simulink model "pulsar_channeliser"  (R2012b)
settings: Solver=ode45  StartTime=0.0  StopTime=450e6  RelTol=1e-3
undefined symbols (not defined in the file): pfb_coeff_gen_calc, sigbuilder_block
libraries: xbsIndex_r4 x10677, casper_library_delays x128, casper_library_misc x45, simulink x17, dspsigops x12, xps_library x9, casper_library_flow_control x4, casper_library_pfbs x2
(part 5 of 105)

== system pulsar_channeliser/frame_counter ==
  note: Knowing the band select will tell us how many
      | channels we actually have to put through,
      | and hence how many words need to be read
      | out of the FIFO at once.
      | Explanation:
      | 0 (16 chans) - 512 words, 64 frames
      | 1 (14 chans) - 518 words, 74 frames
      | 2 (12 chans) - 516 words, 86 frames
      | 3 (10 chans) - 515 words, 103 frames
      | 4 (8 chans) - 512 words, 128 frames
      | 5 (6 chans) - 513 words, 171 frames
      | 6 (4 chans) - 512 words, 256 frames
      | 7 (2 chans) - 512 words, 512 frames
  note: 31-bit counter, along with 10-bit number below, would make a 41-bit
      | output but since the number is 10-bit only to accommodate 512, it'll
      | never actually get to 41 bits. Just 40. So I'll chop the top one off.
  reset : Inport
  dv : Inport  Port=2
  band_select : Inport  Port=3
  Constant10 : xbsIndex_r4/Constant  const=86  gui_display_data_type=Fixed-point  arith_type=Unsigned  n_bits=10  bin_pt=0  preci_type=Single  exp_width=8  frac_width=24  explicit_period=on  period=1  equ=P=C  opselect=C  inp2=PCIN>>17  opr=+  inp1=P  carry=CIN  dbl_ovrd=off  block_type=constant
  Constant11 : xbsIndex_r4/Constant  const=103  gui_display_data_type=Fixed-point  arith_type=Unsigned  n_bits=10  bin_pt=0  preci_type=Single  exp_width=8  frac_width=24  explicit_period=on  period=1  equ=P=C  opselect=C  inp2=PCIN>>17  opr=+  inp1=P  carry=CIN  dbl_ovrd=off  block_type=constant
  Constant12 : xbsIndex_r4/Constant  const=171  gui_display_data_type=Fixed-point  arith_type=Unsigned  n_bits=10  bin_pt=0  preci_type=Single  exp_width=8  frac_width=24  explicit_period=on  period=1  equ=P=C  opselect=C  inp2=PCIN>>17  opr=+  inp1=P  carry=CIN  dbl_ovrd=off  block_type=constant
  Constant13 : xbsIndex_r4/Constant  const=128  gui_display_data_type=Fixed-point  arith_type=Unsigned  n_bits=10  bin_pt=0  preci_type=Single  exp_width=8  frac_width=24  explicit_period=on  period=1  equ=P=C  opselect=C  inp2=PCIN>>17  opr=+  inp1=P  carry=CIN  dbl_ovrd=off  block_type=constant
  Constant14 : xbsIndex_r4/Constant  const=256  gui_display_data_type=Fixed-point  arith_type=Unsigned  n_bits=10  bin_pt=0  preci_type=Single  exp_width=8  frac_width=24  explicit_period=on  period=1  equ=P=C  opselect=C  inp2=PCIN>>17  opr=+  inp1=P  carry=CIN  dbl_ovrd=off  block_type=constant
  Constant15 : xbsIndex_r4/Constant  const=512  gui_display_data_type=Fixed-point  arith_type=Unsigned  n_bits=10  bin_pt=0  preci_type=Single  exp_width=8  frac_width=24  explicit_period=on  period=1  equ=P=C  opselect=C  inp2=PCIN>>17  opr=+  inp1=P  carry=CIN  dbl_ovrd=off  block_type=constant
  Constant7 : xbsIndex_r4/Constant  const=64  gui_display_data_type=Fixed-point  arith_type=Unsigned  n_bits=10  bin_pt=0  preci_type=Single  exp_width=8  frac_width=24  explicit_period=on  period=1  equ=P=C  opselect=C  inp2=PCIN>>17  opr=+  inp1=P  carry=CIN  dbl_ovrd=off  block_type=constant
  Constant9 : xbsIndex_r4/Constant  const=74  gui_display_data_type=Fixed-point  arith_type=Unsigned  n_bits=10  bin_pt=0  preci_type=Single  exp_width=8  frac_width=24  explicit_period=on  period=1  equ=P=C  opselect=C  inp2=PCIN>>17  opr=+  inp1=P  carry=CIN  dbl_ovrd=off  block_type=constant
  Counter : xbsIndex_r4/Counter  cnt_type=Free Running  cnt_to=Inf  operation=Up  start_count=0  cnt_by_val=1  arith_type=Unsigned  n_bits=31  bin_pt=0  load_pin=off  rst=on  en=on  explicit_period=on  period=1  dbl_ovrd=off  use_behavioral_HDL=off  implementation=Fabric  block_type=counter
  Mult : xbsIndex_r4/Mult  precision=Full  arith_type="Signed  (2's comp)"  n_bits=16  bin_pt=14  quantization=Truncate  overflow=Wrap  en=off  latency=3  dbl_ovrd=off  use_behavioral_HDL=off  opt=Speed  use_embedded=on  optimum_pipeline=off  pipeline=on  use_rpm=on  placement_style=Triangular  block_type=mult
  Mux1 : xbsIndex_r4/Mux  inputs=8  en=off  latency=0  precision=Full  arith_type=Unsigned  n_bits=16  bin_pt=14  quantization=Truncate  overflow=Wrap  dbl_ovrd=off  block_type=mux
  Slice : xbsIndex_r4/Slice  nbits=40  boolean_output=off  mode=Lower Bit Location + Width  bit1=0  base1=MSB of Input  bit0=0  base0=LSB of Input  dbl_ovrd=off  block_type=slice
  Slice1 : xbsIndex_r4/Slice  nbits=3  boolean_output=off  mode=Upper Bit Location + Width  bit1=0  base1=MSB of Input  bit0=1  base0=LSB of Input  dbl_ovrd=off  block_type=slice
  edge_detect1 : casper_library_misc/edge_detect  edge=Rising  polarity=Active High  x_in=[0 0.08 0.08 0.16 0.16 0.24 0.24 0.32 0.32 0.4]  y_in="[-1 -1  1  1  1  1  1  1  1  1]"  x_out=[0.6 0.68 0.68 0.76 0.76 0.84 0.84 0.92 0.92 1]  y_out="[-1 -1  1  1 -1 -1 -1 -1 -1 -1]"
  frame_count : Outport
  wires:
  dv/1 -> edge_detect1/1
  reset/1 -> Counter/1
  edge_detect1/1 -> Counter/2
  Slice1/1 -> Mux1/1
  Constant7/1 -> Mux1/2
  Constant9/1 -> Mux1/3
  Constant10/1 -> Mux1/4
  Constant11/1 -> Mux1/5
  Constant12/1 -> Mux1/7
  band_select/1 -> Slice1/1
  Constant13/1 -> Mux1/6
  Constant14/1 -> Mux1/8
  Constant15/1 -> Mux1/9
  Mux1/1 -> Mult/2
  Counter/1 -> Mult/1
  Mult/1 -> Slice/1
  Slice/1 -> frame_count/1

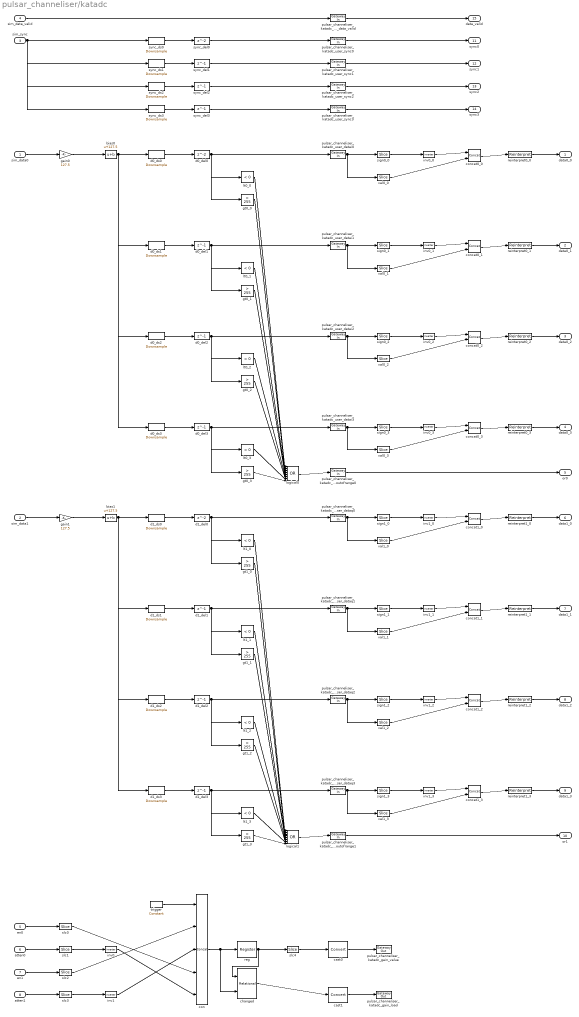
== system pulsar_channeliser/katadc ==
  sim_data0 : Inport
  sim_data1 : Inport  Port=2
  sim_sync : Inport  Port=3
  sim_data_valid : Inport  Port=4
  en0 : Inport  Port=5
  atten0 : Inport  Port=6
  en1 : Inport  Port=7
  atten1 : Inport  Port=8
  bias0 : Bias  Bias=127.5  SaturateOnIntegerOverflow=on
  bias1 : Bias  Bias=127.5  SaturateOnIntegerOverflow=on
  cast0 : xbsIndex_r4/Convert  gui_display_data_type=Fixed-point  arith_type=Unsigned  n_bits=14  bin_pt=0  float_type=Single  exp_bits=8  fraction_bits=24  quantization=Truncate  overflow=Wrap  en=off  latency=0  dbl_ovrd=off  pipeline=off  block_type=convert
      settings: block_version=11.4
  cast1 : xbsIndex_r4/Convert  gui_display_data_type=Fixed-point  arith_type=Boolean  n_bits=16  bin_pt=14  float_type=Single  exp_bits=8  fraction_bits=24  quantization=Truncate  overflow=Wrap  en=off  latency=0  dbl_ovrd=off  pipeline=off  block_type=convert
      settings: block_version=11.4
  changed : xbsIndex_r4/Relational  mode=a!=b  en=off  latency=1  dbl_ovrd=off  block_type=relational
  con : xbsIndex_r4/Concat  num_inputs=5  dbl_ovrd=off  block_type=concat
  concat0_{0..3} (4 alike) : xbsIndex_r4/Concat  num_inputs=2  dbl_ovrd=off  block_type=concat
  concat1_{0..3} (4 alike) : xbsIndex_r4/Concat  num_inputs=2  dbl_ovrd=off  block_type=concat
  d0_del0 : Delay  InputProcessing=Inherited
  d0_del1 : Delay  DelayLength=1  InputProcessing=Inherited
  d0_del2 : Delay  DelayLength=1  InputProcessing=Inherited
  d0_del3 : Delay  DelayLength=1  InputProcessing=Inherited
  d0_ds0 : dspsigops/Downsample  N=4  phase=0  RateOptions=Allow multirate processing  smode=Allow multirate  fmode=Maintain input frame size  ic=0
  d0_ds1 : dspsigops/Downsample  N=4  phase=1  RateOptions=Allow multirate processing  smode=Allow multirate  fmode=Maintain input frame size  ic=0
  d0_ds2 : dspsigops/Downsample  N=4  phase=2  RateOptions=Allow multirate processing  smode=Allow multirate  fmode=Maintain input frame size  ic=0
  d0_ds3 : dspsigops/Downsample  N=4  phase=3  RateOptions=Allow multirate processing  smode=Allow multirate  fmode=Maintain input frame size  ic=0
  d1_del0 : Delay  InputProcessing=Inherited
  d1_del1 : Delay  DelayLength=1  InputProcessing=Inherited
  d1_del2 : Delay  DelayLength=1  InputProcessing=Inherited
  d1_del3 : Delay  DelayLength=1  InputProcessing=Inherited
  d1_ds0 : dspsigops/Downsample  N=4  phase=0  RateOptions=Allow multirate processing  smode=Allow multirate  fmode=Maintain input frame size  ic=0
  d1_ds1 : dspsigops/Downsample  N=4  phase=1  RateOptions=Allow multirate processing  smode=Allow multirate  fmode=Maintain input frame size  ic=0
  d1_ds2 : dspsigops/Downsample  N=4  phase=2  RateOptions=Allow multirate processing  smode=Allow multirate  fmode=Maintain input frame size  ic=0
  d1_ds3 : dspsigops/Downsample  N=4  phase=3  RateOptions=Allow multirate processing  smode=Allow multirate  fmode=Maintain input frame size  ic=0
  gain0 : Gain  Gain=127.5  SaturateOnIntegerOverflow=on  OutDataTypeStr=Inherit: Same as input  ParamDataTypeStr=Inherit: Same as input
  gain1 : Gain  Gain=127.5  SaturateOnIntegerOverflow=on  OutDataTypeStr=Inherit: Same as input  ParamDataTypeStr=Inherit: Same as input
  gt0_{0..3} (4 alike) : simulink/Logic and Bit Operations/Compare To Constant  relop=>  const=255  OutDataTypeStr=boolean  ZeroCross=off
  gt1_{0..3} (4 alike) : simulink/Logic and Bit Operations/Compare To Constant  relop=>  const=255  OutDataTypeStr=boolean  ZeroCross=off
  inv0 : xbsIndex_r4/Inverter  en=off  latency=0  dbl_ovrd=off  block_type=inv
      settings: block_version=11.4
  inv0_{0..3} (4 alike) : xbsIndex_r4/Inverter  en=off  latency=0  dbl_ovrd=off  block_type=inv
      settings: block_version=11.4
  inv1 : xbsIndex_r4/Inverter  en=off  latency=0  dbl_ovrd=off  block_type=inv
      settings: block_version=11.4
  inv1_{0..3} (4 alike) : xbsIndex_r4/Inverter  en=off  latency=0  dbl_ovrd=off  block_type=inv
      settings: block_version=11.4
  logical0 : Logic  Operator=OR  Inputs=8
  logical1 : Logic  Operator=OR  Inputs=8
  lt0_{0..3} (4 alike) : simulink/Logic and Bit Operations/Compare To Constant  relop=<  const=0  OutDataTypeStr=boolean  ZeroCross=off
  lt1_{0..3} (4 alike) : simulink/Logic and Bit Operations/Compare To Constant  relop=<  const=0  OutDataTypeStr=boolean  ZeroCross=off
  pulsar_channeliser_katadc_gain_load : xbsIndex_r4/Gateway Out  inherit_from_input=off  hdl_port=on  timing_constraint=None  locs_specified=off  LOCs={}  UseAsDAC=off  DACChannel='1'  block_type=gatewayout
  pulsar_channeliser_katadc_gain_value : xbsIndex_r4/Gateway Out  inherit_from_input=off  hdl_port=on  timing_constraint=None  locs_specified=off  LOCs={}  UseAsDAC=off  DACChannel='1'  block_type=gatewayout
  pulsar_channeliser_katadc_user_data_valid : xbsIndex_r4/Gateway In  gui_display_data_type=Fixed-point  arith_type=Boolean  n_bits=16  bin_pt=14  preci_type=Single  exp_width=8  frac_width=24  quantization="Round  (unbiased: +/- Inf)"  overflow=Saturate  period=1  dbl_ovrd=off  timing_constraint=None  locs_specified=off  LOCs={}  UseAsADC=off  ADCChannel='1'  inherit_from_input=off  hdl_port=on  block_type=gatewayin
  pulsar_channeliser_katadc_user_datai{0..3} (4 alike) : xbsIndex_r4/Gateway In  gui_display_data_type=Fixed-point  arith_type=Unsigned  n_bits=8  bin_pt=0  preci_type=Single  exp_width=8  frac_width=24  quantization="Round  (unbiased: +/- Inf)"  overflow=Saturate  period=1  dbl_ovrd=off  timing_constraint=None  locs_specified=off  LOCs={}  UseAsADC=off  ADCChannel='1'  inherit_from_input=off  hdl_port=on  block_type=gatewayin
  pulsar_channeliser_katadc_user_dataq{0..3} (4 alike) : xbsIndex_r4/Gateway In  gui_display_data_type=Fixed-point  arith_type=Unsigned  n_bits=8  bin_pt=0  preci_type=Single  exp_width=8  frac_width=24  quantization="Round  (unbiased: +/- Inf)"  overflow=Saturate  period=1  dbl_ovrd=off  timing_constraint=None  locs_specified=off  LOCs={}  UseAsADC=off  ADCChannel='1'  inherit_from_input=off  hdl_port=on  block_type=gatewayin
  pulsar_channeliser_katadc_user_outofrange0 : xbsIndex_r4/Gateway In  gui_display_data_type=Fixed-point  arith_type=Boolean  n_bits=16  bin_pt=14  preci_type=Single  exp_width=8  frac_width=24  quantization="Round  (unbiased: +/- Inf)"  overflow=Saturate  period=1  dbl_ovrd=off  timing_constraint=None  locs_specified=off  LOCs={}  UseAsADC=off  ADCChannel='1'  inherit_from_input=off  hdl_port=on  block_type=gatewayin
  pulsar_channeliser_katadc_user_outofrange1 : xbsIndex_r4/Gateway In  gui_display_data_type=Fixed-point  arith_type=Boolean  n_bits=16  bin_pt=14  preci_type=Single  exp_width=8  frac_width=24  quantization="Round  (unbiased: +/- Inf)"  overflow=Saturate  period=1  dbl_ovrd=off  timing_constraint=None  locs_specified=off  LOCs={}  UseAsADC=off  ADCChannel='1'  inherit_from_input=off  hdl_port=on  block_type=gatewayin
  pulsar_channeliser_katadc_user_sync{0..3} (4 alike) : xbsIndex_r4/Gateway In  gui_display_data_type=Fixed-point  arith_type=Boolean  n_bits=16  bin_pt=14  preci_type=Single  exp_width=8  frac_width=24  quantization="Round  (unbiased: +/- Inf)"  overflow=Saturate  period=1  dbl_ovrd=off  timing_constraint=None  locs_specified=off  LOCs={}  UseAsADC=off  ADCChannel='1'  inherit_from_input=off  hdl_port=on  block_type=gatewayin
  reg : xbsIndex_r4/Register  init=0  rst=off  en=off  dbl_ovrd=off  block_type=register
      settings: block_version=11.4
  reinterpret0_{0..3} (4 alike) : xbsIndex_r4/Reinterpret  force_arith_type=on  arith_type="Signed  (2's comp)"  force_bin_pt=on  bin_pt=7  block_type=reinterpret
      settings: infoedit="Changes signal type without altering the binary representation.   You can changed the signal between signed and unsigned, and relocate the binary point.<br><br>Hardware notes: In hardware this block costs nothing.<br><br>Example:  Suppose the input is 6 bits wide, signed, with 2 fractional bits, and the output is forced to unsigned with 0 fractional bits.  Then an input of -2.0 (1110.00 in binary 2's complement) becomes an output of 56 (111000 in binary)."
  reinterpret1_{0..3} (4 alike) : xbsIndex_r4/Reinterpret  force_arith_type=on  arith_type="Signed  (2's comp)"  force_bin_pt=on  bin_pt=7  block_type=reinterpret
      settings: infoedit="Changes signal type without altering the binary representation.   You can changed the signal between signed and unsigned, and relocate the binary point.<br><br>Hardware notes: In hardware this block costs nothing.<br><br>Example:  Suppose the input is 6 bits wide, signed, with 2 fractional bits, and the output is forced to unsigned with 0 fractional bits.  Then an input of -2.0 (1110.00 in binary 2's complement) becomes an output of 56 (111000 in binary)."
  sign0_{0..3} (4 alike) : xbsIndex_r4/Slice  nbits=1  boolean_output=off  mode=Upper Bit Location + Width  bit1=0  base1=MSB of Input  bit0=0  base0=MSB of Input  dbl_ovrd=off  block_type=slice
  sign1_{0..3} (4 alike) : xbsIndex_r4/Slice  nbits=1  boolean_output=off  mode=Upper Bit Location + Width  bit1=0  base1=MSB of Input  bit0=0  base0=MSB of Input  dbl_ovrd=off  block_type=slice
  slc0 : xbsIndex_r4/Slice  nbits=1  boolean_output=off  mode=Lower Bit Location + Width  bit1=0  base1=MSB of Input  bit0=0  base0=LSB of Input  dbl_ovrd=off  block_type=slice
  slc1 : xbsIndex_r4/Slice  nbits=6  boolean_output=off  mode=Lower Bit Location + Width  bit1=0  base1=MSB of Input  bit0=0  base0=LSB of Input  dbl_ovrd=off  block_type=slice
  slc2 : xbsIndex_r4/Slice  nbits=1  boolean_output=off  mode=Lower Bit Location + Width  bit1=0  base1=MSB of Input  bit0=0  base0=LSB of Input  dbl_ovrd=off  block_type=slice
  slc3 : xbsIndex_r4/Slice  nbits=6  boolean_output=off  mode=Lower Bit Location + Width  bit1=0  base1=MSB of Input  bit0=0  base0=LSB of Input  dbl_ovrd=off  block_type=slice
  slc4 : xbsIndex_r4/Slice  nbits=14  boolean_output=off  mode=Lower Bit Location + Width  bit1=0  base1=MSB of Input  bit0=0  base0=LSB of Input  dbl_ovrd=off  block_type=slice
  sync_del0 : Delay  InputProcessing=Inherited
  sync_del1 : Delay  DelayLength=1  InputProcessing=Inherited
  sync_del2 : Delay  DelayLength=1  InputProcessing=Inherited
  sync_del3 : Delay  DelayLength=1  InputProcessing=Inherited
  sync_ds0 : dspsigops/Downsample  N=4  phase=0  RateOptions=Allow multirate processing  smode=Allow multirate  fmode=Maintain input frame size  ic=0
  sync_ds1 : dspsigops/Downsample  N=4  phase=1  RateOptions=Allow multirate processing  smode=Allow multirate  fmode=Maintain input frame size  ic=0
  sync_ds2 : dspsigops/Downsample  N=4  phase=2  RateOptions=Allow multirate processing  smode=Allow multirate  fmode=Maintain input frame size  ic=0
  sync_ds3 : dspsigops/Downsample  N=4  phase=3  RateOptions=Allow multirate processing  smode=Allow multirate  fmode=Maintain input frame size  ic=0
  trigger : xbsIndex_r4/Constant  const=1  gui_display_data_type=Fixed-point  arith_type=Unsigned  n_bits=1  bin_pt=0  preci_type=Single  exp_width=8  frac_width=24  explicit_period=off  period=1  equ=P=C  opselect=C  inp2=PCIN>>17  opr=+  inp1=P  carry=CIN  dbl_ovrd=off  block_type=constant
      settings: block_version=11.4
  val0_{0..3} (4 alike) : xbsIndex_r4/Slice  nbits=7  boolean_output=off  mode=Lower Bit Location + Width  bit1=0  base1=LSB of Input  bit0=0  base0=LSB of Input  dbl_ovrd=off  block_type=slice
  val1_{0..3} (4 alike) : xbsIndex_r4/Slice  nbits=7  boolean_output=off  mode=Lower Bit Location + Width  bit1=0  base1=LSB of Input  bit0=0  base0=LSB of Input  dbl_ovrd=off  block_type=slice
  data0_0 : Outport
  data0_1 : Outport  Port=2
  data0_2 : Outport  Port=3
  data0_3 : Outport  Port=4
  or0 : Outport  Port=5
  data1_0 : Outport  Port=6
  data1_1 : Outport  Port=7
  data1_2 : Outport  Port=8
  data1_3 : Outport  Port=9
  or1 : Outport  Port=10
  sync0 : Outport  Port=11
  sync1 : Outport  Port=12
  sync2 : Outport  Port=13
  sync3 : Outport  Port=14
  data_valid : Outport  Port=15
  wires:
  sim_data0/1 -> gain0/1
  gain0/1 -> bias0/1
  bias0/1 -> d0_ds0/1, d0_ds1/1, d0_ds2/1, d0_ds3/1
  d0_ds0/1 -> d0_del0/1
  d0_del0/1 -> pulsar_channeliser_katadc_user_datai0/1, lt0_0/1, gt0_0/1
  pulsar_channeliser_katadc_user_datai0/1 -> sign0_0/1, val0_0/1
  sign0_0/1 -> inv0_0/1
  inv0_0/1 -> concat0_0/1
  val0_0/1 -> concat0_0/2
  concat0_0/1 -> reinterpret0_0/1
  reinterpret0_0/1 -> data0_0/1
  d0_ds1/1 -> d0_del1/1
  d0_del1/1 -> pulsar_channeliser_katadc_user_datai1/1, lt0_1/1, gt0_1/1
  pulsar_channeliser_katadc_user_datai1/1 -> sign0_1/1, val0_1/1
  sign0_1/1 -> inv0_1/1
  inv0_1/1 -> concat0_1/1
  val0_1/1 -> concat0_1/2
  concat0_1/1 -> reinterpret0_1/1
  reinterpret0_1/1 -> data0_1/1
  d0_ds2/1 -> d0_del2/1
  d0_del2/1 -> pulsar_channeliser_katadc_user_datai2/1, lt0_2/1, gt0_2/1
  pulsar_channeliser_katadc_user_datai2/1 -> sign0_2/1, val0_2/1
  sign0_2/1 -> inv0_2/1
  inv0_2/1 -> concat0_2/1
  val0_2/1 -> concat0_2/2
  concat0_2/1 -> reinterpret0_2/1
  reinterpret0_2/1 -> data0_2/1
  d0_ds3/1 -> d0_del3/1
  d0_del3/1 -> pulsar_channeliser_katadc_user_datai3/1, lt0_3/1, gt0_3/1
  pulsar_channeliser_katadc_user_datai3/1 -> sign0_3/1, val0_3/1
  sign0_3/1 -> inv0_3/1
  inv0_3/1 -> concat0_3/1
  val0_3/1 -> concat0_3/2
  concat0_3/1 -> reinterpret0_3/1
  reinterpret0_3/1 -> data0_3/1
  lt0_0/1 -> logical0/1
  gt0_0/1 -> logical0/2
  lt0_1/1 -> logical0/3
  gt0_1/1 -> logical0/4
  lt0_2/1 -> logical0/5
  gt0_2/1 -> logical0/6
  lt0_3/1 -> logical0/7
  gt0_3/1 -> logical0/8
  logical0/1 -> pulsar_channeliser_katadc_user_outofrange0/1
  pulsar_channeliser_katadc_user_outofrange0/1 -> or0/1
  sim_data1/1 -> gain1/1
  gain1/1 -> bias1/1
  bias1/1 -> d1_ds0/1, d1_ds1/1, d1_ds2/1, d1_ds3/1
  d1_ds0/1 -> d1_del0/1
  d1_del0/1 -> pulsar_channeliser_katadc_user_dataq0/1, lt1_0/1, gt1_0/1
  pulsar_channeliser_katadc_user_dataq0/1 -> sign1_0/1, val1_0/1
  sign1_0/1 -> inv1_0/1
  inv1_0/1 -> concat1_0/1
  val1_0/1 -> concat1_0/2
  concat1_0/1 -> reinterpret1_0/1
  reinterpret1_0/1 -> data1_0/1
  d1_ds1/1 -> d1_del1/1
  d1_del1/1 -> pulsar_channeliser_katadc_user_dataq1/1, lt1_1/1, gt1_1/1
  pulsar_channeliser_katadc_user_dataq1/1 -> sign1_1/1, val1_1/1
  sign1_1/1 -> inv1_1/1
  inv1_1/1 -> concat1_1/1
  val1_1/1 -> concat1_1/2
  concat1_1/1 -> reinterpret1_1/1
  reinterpret1_1/1 -> data1_1/1
  d1_ds2/1 -> d1_del2/1
  d1_del2/1 -> pulsar_channeliser_katadc_user_dataq2/1, lt1_2/1, gt1_2/1
  pulsar_channeliser_katadc_user_dataq2/1 -> sign1_2/1, val1_2/1
  sign1_2/1 -> inv1_2/1
  inv1_2/1 -> concat1_2/1
  val1_2/1 -> concat1_2/2
  concat1_2/1 -> reinterpret1_2/1
  reinterpret1_2/1 -> data1_2/1
  d1_ds3/1 -> d1_del3/1
  d1_del3/1 -> pulsar_channeliser_katadc_user_dataq3/1, lt1_3/1, gt1_3/1
  pulsar_channeliser_katadc_user_dataq3/1 -> sign1_3/1, val1_3/1
  sign1_3/1 -> inv1_3/1
  inv1_3/1 -> concat1_3/1
  val1_3/1 -> concat1_3/2
  concat1_3/1 -> reinterpret1_3/1
  reinterpret1_3/1 -> data1_3/1
  lt1_0/1 -> logical1/1
  gt1_0/1 -> logical1/2
  lt1_1/1 -> logical1/3
  gt1_1/1 -> logical1/4
  lt1_2/1 -> logical1/5
  gt1_2/1 -> logical1/6
  lt1_3/1 -> logical1/7
  gt1_3/1 -> logical1/8
  logical1/1 -> pulsar_channeliser_katadc_user_outofrange1/1
  pulsar_channeliser_katadc_user_outofrange1/1 -> or1/1
  sim_sync/1 -> sync_ds0/1, sync_ds1/1, sync_ds2/1, sync_ds3/1
  sync_ds0/1 -> sync_del0/1
  sync_del0/1 -> pulsar_channeliser_katadc_user_sync0/1
  pulsar_channeliser_katadc_user_sync0/1 -> sync0/1
  sync_ds1/1 -> sync_del1/1
  sync_del1/1 -> pulsar_channeliser_katadc_user_sync1/1
  pulsar_channeliser_katadc_user_sync1/1 -> sync1/1
  sync_ds2/1 -> sync_del2/1
  sync_del2/1 -> pulsar_channeliser_katadc_user_sync2/1
  pulsar_channeliser_katadc_user_sync2/1 -> sync2/1
  sync_ds3/1 -> sync_del3/1
  sync_del3/1 -> pulsar_channeliser_katadc_user_sync3/1
  pulsar_channeliser_katadc_user_sync3/1 -> sync3/1
  sim_data_valid/1 -> pulsar_channeliser_katadc_user_data_valid/1
  pulsar_channeliser_katadc_user_data_valid/1 -> data_valid/1
  en0/1 -> slc0/1
  atten0/1 -> slc1/1
  slc1/1 -> inv0/1
  en1/1 -> slc2/1
  atten1/1 -> slc3/1
  slc3/1 -> inv1/1
  trigger/1 -> con/1
  slc0/1 -> con/4
  inv0/1 -> con/5
  slc2/1 -> con/2
  inv1/1 -> con/3
  con/1 -> reg/1, changed/2
  reg/1 -> changed/1, slc4/1
  slc4/1 -> cast0/1
  cast0/1 -> pulsar_channeliser_katadc_gain_value/1
  changed/1 -> cast1/1
  cast1/1 -> pulsar_channeliser_katadc_gain_load/1

== system pulsar_channeliser/keep_high_approx_100ms ==
  In1 : Inport
  Counter5 : xbsIndex_r4/Counter  cnt_type=Free Running  cnt_to=Inf  operation=Up  start_count=0  cnt_by_val=1  arith_type=Unsigned  n_bits=26  bin_pt=0  load_pin=off  rst=on  en=on  explicit_period=on  period=1  dbl_ovrd=off  use_behavioral_HDL=off  implementation=Fabric  block_type=counter
  Register3 : xbsIndex_r4/Register  init=0  rst=on  en=on  dbl_ovrd=off  block_type=register
  Slice1 : xbsIndex_r4/Slice  nbits=1  boolean_output=on  mode=Upper Bit Location + Width  bit1=0  base1=MSB of Input  bit0=0  base0=LSB of Input  dbl_ovrd=off  block_type=slice
  edge_detect : casper_library_misc/edge_detect  edge=Rising  polarity=Active High  x_in=[0 0.08 0.08 0.16 0.16 0.24 0.24 0.32 0.32 0.4]  y_in="[-1 -1  1  1  1  1  1  1  1  1]"  x_out=[0.6 0.68 0.68 0.76 0.76 0.84 0.84 0.92 0.92 1]  y_out="[-1 -1  1  1 -1 -1 -1 -1 -1 -1]"
  Out1 : Outport
  wires:
  Counter5/1 -> Slice1/1
  Register3/1 -> Out1/1, Counter5/2
  In1/1 -> edge_detect/1
  Slice1/1 -> Counter5/1, Register3/2
  edge_detect/1 -> Register3/3, Register3/1

== system pulsar_channeliser/latch ==
  set : Inport
  reset : Inport  Port=2
  Register3 : xbsIndex_r4/Register  init=0  rst=on  en=on  dbl_ovrd=off  block_type=register
  out : Outport
  wires:
  Register3/1 -> out/1
  set/1 -> Register3/3, Register3/1
  reset/1 -> Register3/2

== system pulsar_channeliser/latch1 ==
  set : Inport
  reset : Inport  Port=2
  Register3 : xbsIndex_r4/Register  init=0  rst=on  en=on  dbl_ovrd=off  block_type=register
  out : Outport
  wires:
  reset/1 -> Register3/2
  set/1 -> Register3/1, Register3/3
  Register3/1 -> out/1

== system pulsar_channeliser/latch2 ==
  set : Inport
  reset : Inport  Port=2
  Register1 : xbsIndex_r4/Register  init=0  rst=on  en=on  dbl_ovrd=off  block_type=register
  Register3 : xbsIndex_r4/Register  init=0  rst=on  en=on  dbl_ovrd=off  block_type=register
  bus_create2 : Subsystem  AncestorBlock=casper_library_flow_control/bus_create  mask(bus_create){inputNum=2}
      mask prompts: inputNum "Number of inputs:"
      mask init:
      | bus_create_init(gcb,...
      |     'inputNum', inputNum);
  bus_expand9 : Subsystem  AncestorBlock=casper_library_flow_control/bus_expand  mask(bus_expand){mode=divisions of equal size, outputNum=2, outputWidth=1, outputBinaryPt=0, outputArithmeticType=2, show_format=off, outputToWorkspace=off, variablePrefix=out, outputToModelAsWell=on}
      mask prompts: outputNum "Number of outputs:"; outputWidth "Output width:"; outputBinaryPt "Output binary point position:"; outputArithmeticType "Output arithmetic type (ufix=0, fix=1, bool=2):"; show_format "Print format string?"; outputToWorkspace "Output to workspace?"; variablePrefix "Variable name prefix:"; outputToModelAsWell "Output to model as well?"
      mask help:
      | Expands a 'bus' made using a bus_create or Xilinx
      | concat block.
      | The input will be divided into the specified number
      | of outputs with the specified arithmetic types.
      | Divisions are made from most significant bit.
      mask init: same as pulsar_channeliser/bus_expand
      settings: AttributesFormatString=2 outputs
      mask TypeOptions mode: divisions of equal size | divisions of arbitrary size
      mask Callback mode: bus_expand_callback();
      mask Callback outputWidth: bus_expand_callback();
      mask Callback outputToWorkspace: bus_expand_callback();
  out : Outport
  wires:
  reset/1 -> Register1/2, Register3/2
  set/1 -> bus_expand9/1(bus_in)
  bus_expand9/1(msb_out2) -> Register3/3, Register3/1
  bus_expand9/2(lsb_out1) -> Register1/3, Register1/1
  bus_create2/1(bus_out) -> out/1
  Register3/1 -> bus_create2/1(in1)
  Register1/1 -> bus_create2/2(in2)

== system pulsar_channeliser/latch3 ==
  set : Inport
  reset : Inport  Port=2
  Register3 : xbsIndex_r4/Register  init=0  rst=on  en=on  dbl_ovrd=off  block_type=register
  out : Outport
  wires:
  reset/1 -> Register3/2
  set/1 -> Register3/1, Register3/3
  Register3/1 -> out/1

== system pulsar_channeliser/latch4 ==
  set : Inport
  reset : Inport  Port=2
  Register3 : xbsIndex_r4/Register  init=0  rst=on  en=on  dbl_ovrd=off  block_type=register
  out : Outport
  wires:
  Register3/1 -> out/1
  set/1 -> Register3/3, Register3/1
  reset/1 -> Register3/2

== system pulsar_channeliser/latch5 ==
  set : Inport
  reset : Inport  Port=2
  Register3 : xbsIndex_r4/Register  init=0  rst=on  en=on  dbl_ovrd=off  block_type=register
  out : Outport
  wires:
  reset/1 -> Register3/2
  set/1 -> Register3/1, Register3/3
  Register3/1 -> out/1

== system pulsar_channeliser/latch6 ==
  set : Inport
  reset : Inport  Port=2
  Register3 : xbsIndex_r4/Register  init=0  rst=on  en=on  dbl_ovrd=off  block_type=register
  out : Outport
  wires:
  Register3/1 -> out/1
  set/1 -> Register3/3, Register3/1
  reset/1 -> Register3/2

== system pulsar_channeliser/latch7 ==
  set : Inport
  reset : Inport  Port=2
  Register3 : xbsIndex_r4/Register  init=0  rst=on  en=on  dbl_ovrd=off  block_type=register
  out : Outport
  wires:
  reset/1 -> Register3/2
  set/1 -> Register3/1, Register3/3
  Register3/1 -> out/1

== system pulsar_channeliser/latch8 ==
  set : Inport
  reset : Inport  Port=2
  Register3 : xbsIndex_r4/Register  init=0  rst=on  en=on  dbl_ovrd=off  block_type=register
  out : Outport
  wires:
  Register3/1 -> out/1
  set/1 -> Register3/3, Register3/1
  reset/1 -> Register3/2

== system pulsar_channeliser/manual_sync ==
  sim_1 : Inport
  io_delay : xbsIndex_r4/Delay  rst=off  infoeditControl=Selection of Reset will increase slice count due to use of real FFs and instead of SRLs  en=off  latency=0  dbl_ovrd=off  reg_retiming=on  block_type=delay
  pulsar_channeliser_manual_sync_user_data_out : xbsIndex_r4/Gateway In  gui_display_data_type=Fixed-point  arith_type=Unsigned  n_bits=32  bin_pt=0  preci_type=Single  exp_width=8  frac_width=24  quantization="Round  (unbiased: +/- Inf)"  overflow=Saturate  period=1  dbl_ovrd=off  timing_constraint=None  locs_specified=off  LOCs={}  UseAsADC=off  ADCChannel='1'  inherit_from_input=off  hdl_port=on  block_type=gatewayin
  reint1 : xbsIndex_r4/Reinterpret  force_arith_type=on  arith_type=Unsigned  force_bin_pt=on  bin_pt=0  block_type=reinterpret
  slice_reg : xbsIndex_r4/Slice  nbits=32  boolean_output=off  mode=Lower Bit Location + Width  bit1=0  base1=MSB of Input  bit0=0  base0=LSB of Input  dbl_ovrd=off  block_type=slice
  in_reg : Outport
  wires:
  pulsar_channeliser_manual_sync_user_data_out/1 -> io_delay/1
  sim_1/1 -> pulsar_channeliser_manual_sync_user_data_out/1
  io_delay/1 -> slice_reg/1
  slice_reg/1 -> reint1/1
  reint1/1 -> in_reg/1

== system pulsar_channeliser/noise_diode_duty_cycle_en ==
  out_reg : Inport
  assert_reg : xbsIndex_r4/Assert  assert_type=on  type_source=Explicitly  gui_display_data_type=Boolean  arith_type=Boolean  n_bits=1  bin_pt=0  preci_type=Single  exp_width=8  frac_width=24  assert_rate=off  rate_source=Explicitly  period=1  output_port=on  block_type=assert
  cast_gw : xbsIndex_r4/Convert  gui_display_data_type=Fixed-point  arith_type=Unsigned  n_bits=32  bin_pt=0  float_type=Single  exp_bits=8  fraction_bits=24  quantization=Truncate  overflow=Wrap  en=off  latency=0  dbl_ovrd=off  pipeline=off  block_type=convert
  io_delay : xbsIndex_r4/Delay  rst=off  infoeditControl=Selection of Reset will increase slice count due to use of real FFs and instead of SRLs  en=off  latency=0  dbl_ovrd=off  reg_retiming=on  block_type=delay
  pulsar_channeliser_noise_diode_duty_cycle_en_user_data_in : xbsIndex_r4/Gateway Out  inherit_from_input=off  hdl_port=on  timing_constraint=None  locs_specified=off  LOCs={}  UseAsDAC=off  DACChannel='1'  block_type=gatewayout
  reint1 : xbsIndex_r4/Reinterpret  force_arith_type=on  arith_type=Unsigned  force_bin_pt=on  bin_pt=0  block_type=reinterpret
  sim_out : Outport
  wires:
  io_delay/1 -> cast_gw/1
  cast_gw/1 -> pulsar_channeliser_noise_diode_duty_cycle_en_user_data_in/1
  pulsar_channeliser_noise_diode_duty_cycle_en_user_data_in/1 -> sim_out/1
  out_reg/1 -> assert_reg/1
  assert_reg/1 -> reint1/1
  reint1/1 -> io_delay/1

== system pulsar_channeliser/noise_diode_en ==
  out_reg : Inport
  assert_reg : xbsIndex_r4/Assert  assert_type=on  type_source=Explicitly  gui_display_data_type=Boolean  arith_type=Boolean  n_bits=1  bin_pt=0  preci_type=Single  exp_width=8  frac_width=24  assert_rate=off  rate_source=Explicitly  period=1  output_port=on  block_type=assert
  cast_gw : xbsIndex_r4/Convert  gui_display_data_type=Fixed-point  arith_type=Unsigned  n_bits=32  bin_pt=0  float_type=Single  exp_bits=8  fraction_bits=24  quantization=Truncate  overflow=Wrap  en=off  latency=0  dbl_ovrd=off  pipeline=off  block_type=convert
  io_delay : xbsIndex_r4/Delay  rst=off  infoeditControl=Selection of Reset will increase slice count due to use of real FFs and instead of SRLs  en=off  latency=0  dbl_ovrd=off  reg_retiming=on  block_type=delay
  pulsar_channeliser_noise_diode_en_user_data_in : xbsIndex_r4/Gateway Out  inherit_from_input=off  hdl_port=on  timing_constraint=None  locs_specified=off  LOCs={}  UseAsDAC=off  DACChannel='1'  block_type=gatewayout
  reint1 : xbsIndex_r4/Reinterpret  force_arith_type=on  arith_type=Unsigned  force_bin_pt=on  bin_pt=0  block_type=reinterpret
  sim_out : Outport
  wires:
  io_delay/1 -> cast_gw/1
  cast_gw/1 -> pulsar_channeliser_noise_diode_en_user_data_in/1
  pulsar_channeliser_noise_diode_en_user_data_in/1 -> sim_out/1
  out_reg/1 -> assert_reg/1
  assert_reg/1 -> reint1/1
  reint1/1 -> io_delay/1

== system pulsar_channeliser/noise_diode_off_length ==
  out_reg : Inport
  assert_reg : xbsIndex_r4/Assert  assert_type=on  type_source=Explicitly  gui_display_data_type=Fixed-point  arith_type=Unsigned  n_bits=32  bin_pt=0  preci_type=Single  exp_width=8  frac_width=24  assert_rate=off  rate_source=Explicitly  period=1  output_port=on  block_type=assert
  cast_gw : xbsIndex_r4/Convert  gui_display_data_type=Fixed-point  arith_type=Unsigned  n_bits=32  bin_pt=0  float_type=Single  exp_bits=8  fraction_bits=24  quantization=Truncate  overflow=Wrap  en=off  latency=0  dbl_ovrd=off  pipeline=off  block_type=convert
  io_delay : xbsIndex_r4/Delay  rst=off  infoeditControl=Selection of Reset will increase slice count due to use of real FFs and instead of SRLs  en=off  latency=0  dbl_ovrd=off  reg_retiming=on  block_type=delay
  pulsar_channeliser_noise_diode_off_length_user_data_in : xbsIndex_r4/Gateway Out  inherit_from_input=off  hdl_port=on  timing_constraint=None  locs_specified=off  LOCs={}  UseAsDAC=off  DACChannel='1'  block_type=gatewayout
  reint1 : xbsIndex_r4/Reinterpret  force_arith_type=on  arith_type=Unsigned  force_bin_pt=on  bin_pt=0  block_type=reinterpret
  sim_out : Outport
  wires:
  io_delay/1 -> cast_gw/1
  cast_gw/1 -> pulsar_channeliser_noise_diode_off_length_user_data_in/1
  pulsar_channeliser_noise_diode_off_length_user_data_in/1 -> sim_out/1
  out_reg/1 -> assert_reg/1
  assert_reg/1 -> reint1/1
  reint1/1 -> io_delay/1

== system pulsar_channeliser/noise_diode_on_length ==
  out_reg : Inport
  assert_reg : xbsIndex_r4/Assert  assert_type=on  type_source=Explicitly  gui_display_data_type=Fixed-point  arith_type=Unsigned  n_bits=32  bin_pt=0  preci_type=Single  exp_width=8  frac_width=24  assert_rate=off  rate_source=Explicitly  period=1  output_port=on  block_type=assert
  cast_gw : xbsIndex_r4/Convert  gui_display_data_type=Fixed-point  arith_type=Unsigned  n_bits=32  bin_pt=0  float_type=Single  exp_bits=8  fraction_bits=24  quantization=Truncate  overflow=Wrap  en=off  latency=0  dbl_ovrd=off  pipeline=off  block_type=convert
  io_delay : xbsIndex_r4/Delay  rst=off  infoeditControl=Selection of Reset will increase slice count due to use of real FFs and instead of SRLs  en=off  latency=0  dbl_ovrd=off  reg_retiming=on  block_type=delay
  pulsar_channeliser_noise_diode_on_length_user_data_in : xbsIndex_r4/Gateway Out  inherit_from_input=off  hdl_port=on  timing_constraint=None  locs_specified=off  LOCs={}  UseAsDAC=off  DACChannel='1'  block_type=gatewayout
  reint1 : xbsIndex_r4/Reinterpret  force_arith_type=on  arith_type=Unsigned  force_bin_pt=on  bin_pt=0  block_type=reinterpret
  sim_out : Outport
  wires:
  io_delay/1 -> cast_gw/1
  cast_gw/1 -> pulsar_channeliser_noise_diode_on_length_user_data_in/1
  pulsar_channeliser_noise_diode_on_length_user_data_in/1 -> sim_out/1
  out_reg/1 -> assert_reg/1
  assert_reg/1 -> reint1/1
  reint1/1 -> io_delay/1

== system pulsar_channeliser/overflows ==
  out_adc0or : Inport
  out_adc1or : Inport  Port=2
  out_fftof : Inport  Port=3
  out_rq0of : Inport  Port=4
  out_rq1of : Inport  Port=5
  out_sp0of : Inport  Port=6
  out_sp1of : Inport  Port=7
  out_tx0of : Inport  Port=8
  out_tx1of : Inport  Port=9
  assert_adc0or : xbsIndex_r4/Assert  assert_type=on  type_source=Explicitly  gui_display_data_type=Boolean  arith_type=Boolean  n_bits=1  bin_pt=0  preci_type=Single  exp_width=8  frac_width=24  assert_rate=off  rate_source=Explicitly  period=1  output_port=on  block_type=assert
  assert_adc1or : xbsIndex_r4/Assert  assert_type=on  type_source=Explicitly  gui_display_data_type=Boolean  arith_type=Boolean  n_bits=1  bin_pt=0  preci_type=Single  exp_width=8  frac_width=24  assert_rate=off  rate_source=Explicitly  period=1  output_port=on  block_type=assert
  assert_fftof : xbsIndex_r4/Assert  assert_type=on  type_source=Explicitly  gui_display_data_type=Fixed-point  arith_type=Unsigned  n_bits=2  bin_pt=0  preci_type=Single  exp_width=8  frac_width=24  assert_rate=off  rate_source=Explicitly  period=1  output_port=on  block_type=assert
  assert_rq0of : xbsIndex_r4/Assert  assert_type=on  type_source=Explicitly  gui_display_data_type=Boolean  arith_type=Boolean  n_bits=1  bin_pt=0  preci_type=Single  exp_width=8  frac_width=24  assert_rate=off  rate_source=Explicitly  period=1  output_port=on  block_type=assert
  assert_rq1of : xbsIndex_r4/Assert  assert_type=on  type_source=Explicitly  gui_display_data_type=Boolean  arith_type=Boolean  n_bits=1  bin_pt=0  preci_type=Single  exp_width=8  frac_width=24  assert_rate=off  rate_source=Explicitly  period=1  output_port=on  block_type=assert
  assert_sp0of : xbsIndex_r4/Assert  assert_type=on  type_source=Explicitly  gui_display_data_type=Boolean  arith_type=Boolean  n_bits=1  bin_pt=0  preci_type=Single  exp_width=8  frac_width=24  assert_rate=off  rate_source=Explicitly  period=1  output_port=on  block_type=assert
  assert_sp1of : xbsIndex_r4/Assert  assert_type=on  type_source=Explicitly  gui_display_data_type=Boolean  arith_type=Boolean  n_bits=1  bin_pt=0  preci_type=Single  exp_width=8  frac_width=24  assert_rate=off  rate_source=Explicitly  period=1  output_port=on  block_type=assert
  assert_tx0of : xbsIndex_r4/Assert  assert_type=on  type_source=Explicitly  gui_display_data_type=Boolean  arith_type=Boolean  n_bits=1  bin_pt=0  preci_type=Single  exp_width=8  frac_width=24  assert_rate=off  rate_source=Explicitly  period=1  output_port=on  block_type=assert
  assert_tx1of : xbsIndex_r4/Assert  assert_type=on  type_source=Explicitly  gui_display_data_type=Boolean  arith_type=Boolean  n_bits=1  bin_pt=0  preci_type=Single  exp_width=8  frac_width=24  assert_rate=off  rate_source=Explicitly  period=1  output_port=on  block_type=assert
  cast_gw : xbsIndex_r4/Convert  gui_display_data_type=Fixed-point  arith_type=Unsigned  n_bits=32  bin_pt=0  float_type=Single  exp_bits=8  fraction_bits=24  quantization=Truncate  overflow=Wrap  en=off  latency=0  dbl_ovrd=off  pipeline=off  block_type=convert
  concatenate : xbsIndex_r4/Concat  num_inputs=9  dbl_ovrd=off  block_type=concat
  io_delay : xbsIndex_r4/Delay  rst=off  infoeditControl=Selection of Reset will increase slice count due to use of real FFs and instead of SRLs  en=off  latency=0  dbl_ovrd=off  reg_retiming=on  block_type=delay
  pulsar_channeliser_overflows_user_data_in : xbsIndex_r4/Gateway Out  inherit_from_input=off  hdl_port=on  timing_constraint=None  locs_specified=off  LOCs={}  UseAsDAC=off  DACChannel='1'  block_type=gatewayout
  reint{1..9} (9 alike) : xbsIndex_r4/Reinterpret  force_arith_type=on  arith_type=Unsigned  force_bin_pt=on  bin_pt=0  block_type=reinterpret
  sim_out : Outport
  wires:
  concatenate/1 -> io_delay/1
  io_delay/1 -> cast_gw/1
  cast_gw/1 -> pulsar_channeliser_overflows_user_data_in/1
  pulsar_channeliser_overflows_user_data_in/1 -> sim_out/1
  out_adc0or/1 -> assert_adc0or/1
  assert_adc0or/1 -> reint1/1
  reint1/1 -> concatenate/1
  out_adc1or/1 -> assert_adc1or/1
  assert_adc1or/1 -> reint2/1
  reint2/1 -> concatenate/2
  out_fftof/1 -> assert_fftof/1
  assert_fftof/1 -> reint3/1
  reint3/1 -> concatenate/3
  out_rq0of/1 -> assert_rq0of/1
  assert_rq0of/1 -> reint4/1
  reint4/1 -> concatenate/4
  out_rq1of/1 -> assert_rq1of/1
  assert_rq1of/1 -> reint5/1
  reint5/1 -> concatenate/5
  out_sp0of/1 -> assert_sp0of/1
  assert_sp0of/1 -> reint6/1
  reint6/1 -> concatenate/6
  out_sp1of/1 -> assert_sp1of/1
  assert_sp1of/1 -> reint7/1
  reint7/1 -> concatenate/7
  out_tx0of/1 -> assert_tx0of/1
  assert_tx0of/1 -> reint8/1
  reint8/1 -> concatenate/8
  out_tx1of/1 -> assert_tx1of/1
  assert_tx1of/1 -> reint9/1
  reint9/1 -> concatenate/9

== system pulsar_channeliser/packetiser_snap ==
  in_word : Inport
  we : Inport  Port=2
  trig : Inport  Port=3
  assert_word : xbsIndex_r4/Assert  assert_type=on  type_source=Explicitly  gui_display_data_type=Fixed-point  arith_type=Unsigned  n_bits=64  bin_pt=0  preci_type=Single  exp_width=8  frac_width=24  assert_rate=off  rate_source=Explicitly  period=1  output_port=on  block_type=assert
  buscreate : Subsystem  AncestorBlock=casper_library_flow_control/bus_create  mask(bus_create){inputNum=1}
      mask prompts: inputNum "Number of inputs:"
      mask init:
      | bus_create_init(gcb,...
      |     'inputNum', inputNum);
  ss : Subsystem  Tag=casper:snapshot  AncestorBlock=casper_library_scopes/snapshot  mask(snapshot){storage=bram, dram_dimm=2, dram_clock=250, nsamples=10, data_width=64, offset=off, circap=off, value=off, use_dsp48=on}
      mask prompts: storage "Storage medium"; dram_dimm "DRAM dimm"; dram_clock "DRAM clock rate"; nsamples "Number of Samples (2^?)"; data_width "Data width"; offset "Start delay support"; circap "Circular capture support"; value "Extra value capture support"; use_dsp48 "Use DSP48s to implement counters"
      mask help:
      | Standard snap block, but with the following optional extras;
      |  1) Optionally delay the fabric trigger by a user-specified number of valids.
      |  2) Capture continuously after a trigger until a stop pulse is received. Data is captured into BRAM continuously, with old data being overwritten until a stop command is received. Then stop capturing when memory is filled. This enables you to get some data before and some data after the stop pulse. Use the 'tr_en_cnt' register to determine where you are in your vector. 'Addr' register's MSb now indicates 'busy capturing'.
      |  3) Optionally capture a value on an input port to a register at the same time as the first data sample.
      |  4) Implement counters using DSP48Es to save resources.
      mask init: same as pulsar_channeliser/acc_snap/ss
      mask TypeOptions storage: bram | dram
      mask Callback storage: snapshot_callback();
      mask TypeOptions dram_dimm: 1 | 2 | 3 | 4
      mask TypeOptions dram_clock: 200 | 250 | 266 | 300 | 333
      mask TypeOptions data_width: 8 | 16 | 32 | 64 | 128
  wires:
  buscreate/1(bus_out) -> ss/1(din)
  in_word/1 -> assert_word/1
  assert_word/1 -> buscreate/1(in1)
  we/1 -> ss/2(we)
  trig/1 -> ss/3(trig)

== system pulsar_channeliser/packetizer ==
  din_valid : Inport
  din : Inport  Port=2
  reset : Inport  Port=3
  Counter : xbsIndex_r4/Counter  cnt_type=Free Running  cnt_to=Inf  operation=Up  start_count=0  cnt_by_val=1  arith_type=Unsigned  n_bits=11  bin_pt=0  load_pin=off  rst=on  en=on  explicit_period=on  period=1  dbl_ovrd=off  use_behavioral_HDL=off  implementation=Fabric  use_rpm=off  block_type=counter
  Inverter : xbsIndex_r4/Inverter  en=off  latency=0  dbl_ovrd=off  block_type=inv
  Logical : xbsIndex_r4/Logical  logical_function=AND  inputs=2  en=off  latency=0  precision=Full  arith_type=Unsigned  n_bits=16  bin_pt=0  align_bp=on  dbl_ovrd=off  block_type=logical
  Logical1 : xbsIndex_r4/Logical  logical_function=AND  inputs=2  en=off  latency=0  precision=Full  arith_type=Unsigned  n_bits=16  bin_pt=0  align_bp=on  dbl_ovrd=off  block_type=logical
  control_fsm : xbsIndex_r4/MCode  mfname=packetizer_fsm  explicit_period=on  period=1  inputsTable={'boundInpExpr'=>['','','3','',' 2047 ',''],'inputs'=>['fifo_empty','shift_count','data_per_word','data_count','n_words','reset']}  outputsTable={'outputs'=>['fifo_re','bram_addr_en','bram_we','serializer_shift','serializer_ld','shift_count_en','shift_count_rst','bram_addr_rst','data_count_en','data_count_rst','done'],'suppressOut'=>['off','off','off','off','off','off','off','off','off','off','off']}  dbl_ovrd=off  enable_stdout=off  enable_debug=off  suppress_output=1  defparams={'data_per_word',3,'n_words', 2047 }  hide_port_list={}  block_type=mcode
      settings: block_version=10.1.3
  data_buffer : xbsIndex_r4/FIFO  mem_type=Block RAM  performance_options=Standard_FIFO  infoedit1=Available only for V4, V5, V6, V7, K7, A7 and Zynq devices.  embedded_registers=off  depth=1K  percent_nbits=8  rst=on  en=off  use_dcount=off  use_percent_full_port=on  use_almost_empty=off  almost_empty_thresh=2  use_almost_full=off  almost_full_thresh=14  dbl_ovrd=off  explicit_period=off  block_type=fifo
      settings: block_version=10.1.3
  data_counter : xbsIndex_r4/Counter  cnt_type=Free Running  cnt_to=Inf  operation=Up  start_count=0  cnt_by_val=1  arith_type=Unsigned  n_bits=12  bin_pt=0  load_pin=off  rst=on  en=on  explicit_period=on  period=1  dbl_ovrd=off  use_behavioral_HDL=off  implementation=Fabric  use_rpm=off  block_type=counter
  parallel_to_serial_converter : Subsystem  AncestorBlock=casper_library_flow_control/parallel_to_serial_converter  mask(parallel_to_serial_converter){pin_width=256, sout_width=64}
      mask prompts: pin_width "Parallel Input Width"; sout_width "Serial Output Width"
      mask help:
      | This block takes as input a parallel bus of specified width.
      | When the load signal 'ld' is asserted, this data is broken into
      | pieces of width specified by the serial output width and
      | stored into different registers chained to form a shift register.
      | If the 'shift' input is subsequently asserted, the shift register
      | returns as output a new piece of data of width sout_width.  This data
      | is the next least significant piece of the original bus.  The converter
      | serializes SMALL ENDIAN.
      |
      | Note that the load operation automatically loads the least significant
      | bits into the register closest to the output, so the first 'shift'
      | assertion changes the data output from bits [sout_width-1:0] to
      | bits [2*sout_width-1:sout_width].
      mask init:
      | parallel_to_serial_converter_init(gcb, ...
      |     'pin_width', pin_width, ...
      |     'sout_width', sout_width);
  shift_counter : xbsIndex_r4/Counter  cnt_type=Free Running  cnt_to=Inf  operation=Up  start_count=0  cnt_by_val=1  arith_type=Unsigned  n_bits=3  bin_pt=0  load_pin=off  rst=on  en=on  explicit_period=on  period=1  dbl_ovrd=off  use_behavioral_HDL=off  implementation=Fabric  use_rpm=off  block_type=counter
  data_addr : Outport
  data_sout : Outport  Port=2
  data_valid : Outport  Port=3
  buffer_overflow : Outport  Port=4
  perc_full : Outport  Port=5
  done : Outport  Port=6
  wires:
  control_fsm/11 -> done/1
  data_buffer/3 -> perc_full/1
  Logical1/1 -> buffer_overflow/1
  data_buffer/4 -> Logical1/2, Inverter/1
  Inverter/1 -> Logical/2
  din_valid/1 -> Logical1/1, Logical/1
  Logical/1 -> data_buffer/2
  data_buffer/1 -> parallel_to_serial_converter/1(pin)
  control_fsm/1 -> data_buffer/3
  control_fsm/4 -> parallel_to_serial_converter/3(shift)
  control_fsm/5 -> parallel_to_serial_converter/2(ld)
  control_fsm/3 -> data_valid/1
  din/1 -> data_buffer/1
  parallel_to_serial_converter/1(sout) -> data_sout/1
  control_fsm/6 -> shift_counter/2
  shift_counter/1 -> control_fsm/2
  control_fsm/7 -> shift_counter/1
  data_buffer/2 -> control_fsm/1
  Counter/1 -> data_addr/1
  control_fsm/2 -> Counter/2
  control_fsm/8 -> Counter/1
  control_fsm/9 -> data_counter/2
  data_counter/1 -> control_fsm/3
  reset/1 -> control_fsm/4, data_buffer/4
  control_fsm/10 -> data_counter/1
